simulink model "psk_demodulate_block1"  (R2020b)
settings: Solver=FixedStepDiscrete  StartTime=0.0  StopTime=10.0  RelTol=1e-3
settings Model: DataTypeOverride=Off  Creator=wardo  LastModifiedBy=wardo
settings DataIOCC: LimitDataPoints=on  SaveOutput=off  SaveTime=off
settings OptimizationCC: BlockReduction=off  ConditionallyExecuteInputs=off  DefaultParameterBehavior=Inlined  LifeSpan=inf
settings DebuggingCC: AlgebraicLoopMsg=error  SingleTaskRateTransMsg=error  AllowSymbolicDim=off  StrictBusMsg=ErrorOnBusTreatedAsVector  SFUnexpectedBacktrackingDiag=warning  SFNoUnconditionalDefaultTransitionDiag=warning  SFExecutionAtInitializationDiag=none  ArithmeticOperatorsInVariantConditions=warning
settings HardwareCC: ProdBitPerPointer=32  ProdBitPerSizeT=32  ProdBitPerPtrDiffT=32  ProdLargestAtomicFloat=None  ProdIntDivRoundTo=Undefined  ProdEndianess=Unspecified  ProdWordSize=32  ProdHWDeviceType=ASIC/FPGA->ASIC/FPGA  ProdEqTarget=off
settings SFSimCC: SimUseLocalCustomCode=off  CustomCodeUndefinedFunction=UseInterfaceOnly
settings RTWCC: RTWUseLocalCustomCode=off
settings CodeAppCC: StateflowObjectComments=on
settings GRTTargetCC: TargetLangStandard=C89/C90 (ANSI)
settings ConfigComp: CovScope=ReferencedModels  CovMetricSettings=dw  CovSaveCumulativeToWorkspaceVar=on  CovSaveSingleToWorkspaceVar=on  CovExternalEMLEnable=off  CovSFcnEnable=off

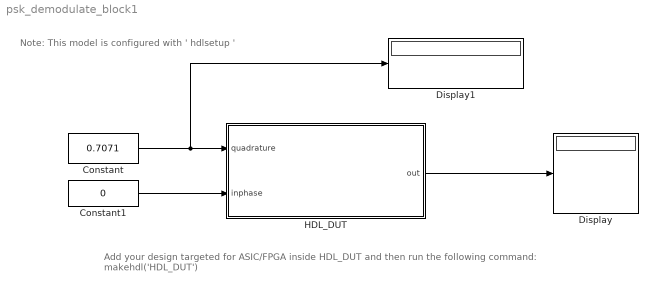
== system psk_demodulate_block1 ==
  note: Note: This model is configured with ' hdlsetup '
  note: Add your design targeted for ASIC/FPGA inside HDL_DUT and then run the following command:
      | makehdl('HDL_DUT')
  Constant : Constant  Value=0.7071  OutDataTypeStr=single  SampleTime=-1
  Constant1 : Constant  Value=0  OutDataTypeStr=single  SampleTime=-1
  Display : Display
  Display1 : Display
  HDL_DUT : Subsystem
  wires:
  Constant/1 -> Display1/1, HDL_DUT/1(quadrature)
  HDL_DUT/1(out) -> Display/1
  Constant1/1 -> HDL_DUT/2(inphase)

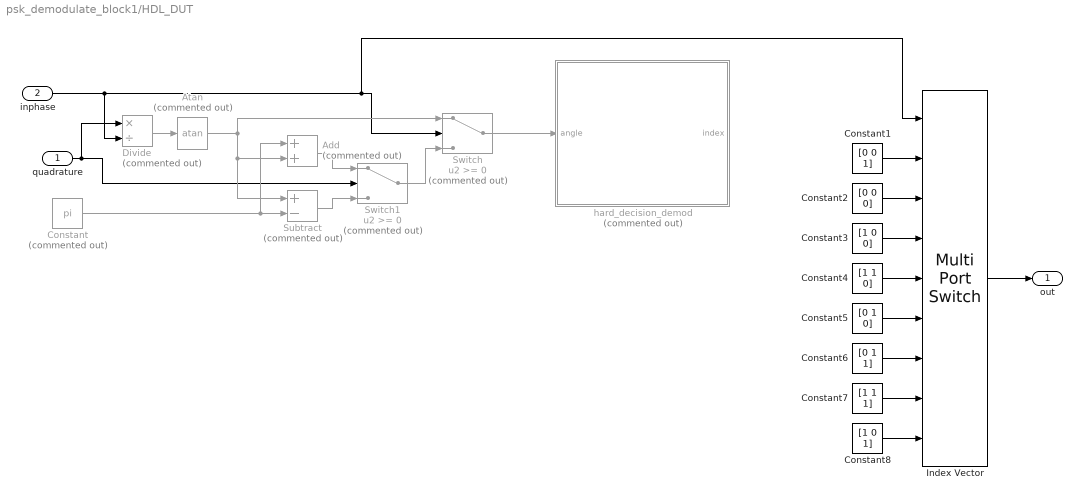
== system psk_demodulate_block1/HDL_DUT ==
  quadrature : Inport
  inphase : Inport  Port=2
  Add : Sum  Commented=on
  Atan : Trigonometry  Commented=on  Operator=atan  ApproximationMethod=CORDIC  OutputSignalType=real
  Constant : Constant  Commented=on  Value=pi  OutDataTypeStr=single  SampleTime=-1
  Constant1 : Constant  Value=[0 0 1]  OutDataTypeStr=single  SampleTime=-1
  Constant2 : Constant  Value=[0 0 0]  OutDataTypeStr=single  SampleTime=-1
  Constant3 : Constant  Value=[1 0 0]  OutDataTypeStr=single  SampleTime=-1
  Constant4 : Constant  Value=[1 1 0]  OutDataTypeStr=single  SampleTime=-1
  Constant5 : Constant  Value=[0 1 0]  OutDataTypeStr=single  SampleTime=-1
  Constant6 : Constant  Value=[0 1 1]  OutDataTypeStr=single  SampleTime=-1
  Constant7 : Constant  Value=[1 1 1]  OutDataTypeStr=single  SampleTime=-1
  Constant8 : Constant  Value=[1 0 1]  OutDataTypeStr=single  SampleTime=-1
  Divide : Product  Commented=on  Inputs=*/  SaturateOnIntegerOverflow=on
  Index Vector : MultiPortSwitch  Inputs=8  DataPortIndices={1,2,3,4,5,6,7,8}  DiagnosticForDefault=Warning  OutDataTypeStr=single
  Subtract : Sum  Commented=on  Inputs=+-
  Switch : Switch  Commented=on
  Switch1 : Switch  Commented=on
  hard_decision_demod : Subsystem  Commented=on
  out : Outport  VectorParamsAs1DForOutWhenUnconnected=off
  wires:
  Divide/1 -> Atan/1
  quadrature/1 -> Divide/1, Switch1/2
  inphase/1 -> Divide/2, Index Vector/1, Switch/2
  Atan/1 -> Add/2, Subtract/1, Switch/1
  Switch1/1 -> Switch/3
  Constant/1 -> Add/1, Subtract/2
  Add/1 -> Switch1/1
  Subtract/1 -> Switch1/3
  Index Vector/1 -> out/1
  Switch/1 -> hard_decision_demod/1(angle)
  Constant1/1 -> Index Vector/2
  Constant2/1 -> Index Vector/3
  Constant4/1 -> Index Vector/5
  Constant3/1 -> Index Vector/4
  Constant8/1 -> Index Vector/9
  Constant6/1 -> Index Vector/7
  Constant7/1 -> Index Vector/8
  Constant5/1 -> Index Vector/6

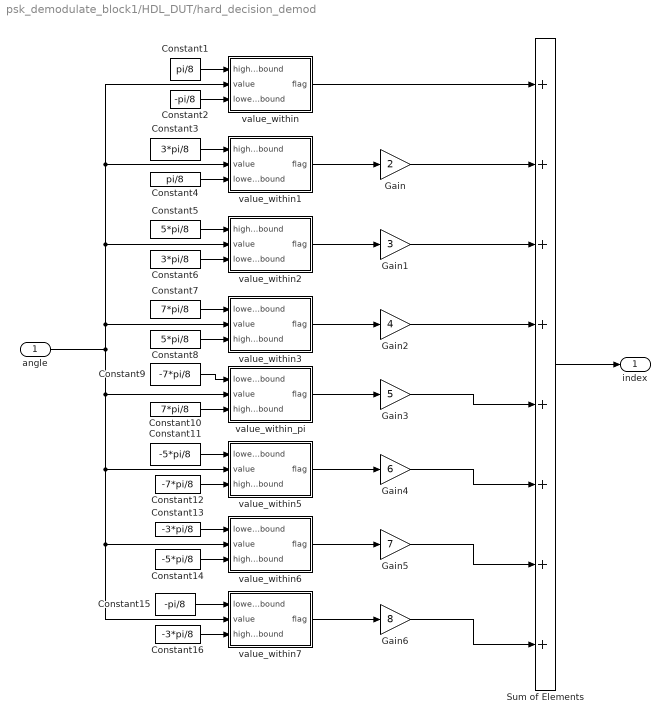
== system psk_demodulate_block1/HDL_DUT/hard_decision_demod ==
  angle : Inport
  Constant1 : Constant  Value=pi/8  OutDataTypeStr=single  SampleTime=-1
  Constant10 : Constant  Value=7*pi/8  OutDataTypeStr=single  SampleTime=-1
  Constant11 : Constant  Value=-5*pi/8  OutDataTypeStr=single  SampleTime=-1
  Constant12 : Constant  Value=-7*pi/8  OutDataTypeStr=single  SampleTime=-1
  Constant13 : Constant  Value=-3*pi/8  OutDataTypeStr=single  SampleTime=-1
  Constant14 : Constant  Value=-5*pi/8  OutDataTypeStr=single  SampleTime=-1
  Constant15 : Constant  Value=-pi/8  OutDataTypeStr=single  SampleTime=-1
  Constant16 : Constant  Value=-3*pi/8  OutDataTypeStr=single  SampleTime=-1
  Constant2 : Constant  Value=-pi/8  OutDataTypeStr=single  SampleTime=-1
  Constant3 : Constant  Value=3*pi/8  OutDataTypeStr=single  SampleTime=-1
  Constant4 : Constant  Value=pi/8  OutDataTypeStr=single  SampleTime=-1
  Constant5 : Constant  Value=5*pi/8  OutDataTypeStr=single  SampleTime=-1
  Constant6 : Constant  Value=3*pi/8  OutDataTypeStr=single  SampleTime=-1
  Constant7 : Constant  Value=7*pi/8  OutDataTypeStr=single  SampleTime=-1
  Constant8 : Constant  Value=5*pi/8  OutDataTypeStr=single  SampleTime=-1
  Constant9 : Constant  Value=-7*pi/8  OutDataTypeStr=single  SampleTime=-1
  Gain : Gain  Gain=2
  Gain1 : Gain  Gain=3
  Gain2 : Gain  Gain=4
  Gain3 : Gain  Gain=5
  Gain4 : Gain  Gain=6
  Gain5 : Gain  Gain=7
  Gain6 : Gain  Gain=8
  Sum of Elements : Sum  Inputs=++++++++
  value_within : Subsystem  TreatAsAtomicUnit=on
  value_within1 : Subsystem  TreatAsAtomicUnit=on
  value_within2 : Subsystem  TreatAsAtomicUnit=on
  value_within3 : Subsystem  TreatAsAtomicUnit=on
  value_within5 : Subsystem  TreatAsAtomicUnit=on
  value_within6 : Subsystem  TreatAsAtomicUnit=on
  value_within7 : Subsystem  TreatAsAtomicUnit=on
  value_within_pi : Subsystem  TreatAsAtomicUnit=on
  index : Outport
  wires:
  Constant2/1 -> value_within/3(lower_bound)
  Constant1/1 -> value_within/1(higher_bound)
  Sum of Elements/1 -> index/1
  Constant3/1 -> value_within1/1(higher_bound)
  Constant4/1 -> value_within1/3(lower_bound)
  Constant5/1 -> value_within2/1(higher_bound)
  Constant7/1 -> value_within3/1(lower_bound)
  Constant6/1 -> value_within2/3(lower_bound)
  Constant13/1 -> value_within6/1(lower_bound)
  Constant9/1 -> value_within_pi/1(lower_bound)
  Constant15/1 -> value_within7/1(lower_bound)
  Constant16/1 -> value_within7/3(higher_bound)
  Constant12/1 -> value_within5/3(higher_bound)
  Constant11/1 -> value_within5/1(lower_bound)
  Constant14/1 -> value_within6/3(higher_bound)
  Constant10/1 -> value_within_pi/3(higher_bound)
  angle/1 -> value_within1/2(value), value_within/2(value), value_within2/2(value), value_within3/2(value), value_within7/2(value), value_within6/2(value), value_within5/2(value), value_within_pi/2(value)
  value_within5/1(flag) -> Gain4/1
  value_within6/1(flag) -> Gain5/1
  value_within7/1(flag) -> Gain6/1
  value_within3/1(flag) -> Gain2/1
  value_within1/1(flag) -> Gain/1
  value_within/1(flag) -> Sum of Elements/1
  Gain/1 -> Sum of Elements/2
  value_within2/1(flag) -> Gain1/1
  Gain1/1 -> Sum of Elements/3
  Gain2/1 -> Sum of Elements/4
  value_within_pi/1(flag) -> Gain3/1
  Gain3/1 -> Sum of Elements/5
  Gain5/1 -> Sum of Elements/7
  Gain6/1 -> Sum of Elements/8
  Gain4/1 -> Sum of Elements/6
  Constant8/1 -> value_within3/3(higher_bound)

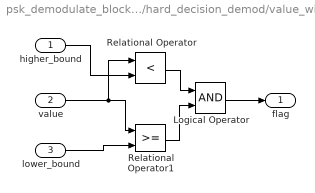
== system psk_demodulate_block1/HDL_DUT/hard_decision_demod/value_within ==
  higher_bound : Inport
  value : Inport  Port=2
  lower_bound : Inport  Port=3
  Logical Operator : Logic  AllPortsSameDT=off  OutDataTypeStr=boolean
  Relational Operator : RelationalOperator  Operator=<  OutDataTypeStr=boolean  RndMeth=Nearest
  Relational Operator1 : RelationalOperator  OutDataTypeStr=boolean  RndMeth=Nearest
  flag : Outport
  wires:
  value/1 -> Relational Operator/1, Relational Operator1/1
  Relational Operator/1 -> Logical Operator/1
  lower_bound/1 -> Relational Operator1/2
  Relational Operator1/1 -> Logical Operator/2
  Logical Operator/1 -> flag/1
  higher_bound/1 -> Relational Operator/2

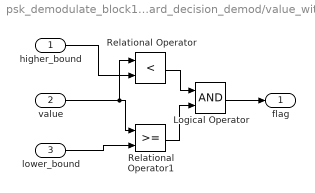
== system psk_demodulate_block1/HDL_DUT/hard_decision_demod/value_within1 ==
  higher_bound : Inport
  value : Inport  Port=2
  lower_bound : Inport  Port=3
  Logical Operator : Logic  AllPortsSameDT=off  OutDataTypeStr=boolean
  Relational Operator : RelationalOperator  Operator=<  OutDataTypeStr=boolean  RndMeth=Nearest
  Relational Operator1 : RelationalOperator  OutDataTypeStr=boolean  RndMeth=Nearest
  flag : Outport
  wires:
  value/1 -> Relational Operator/1, Relational Operator1/1
  Relational Operator/1 -> Logical Operator/1
  lower_bound/1 -> Relational Operator1/2
  Relational Operator1/1 -> Logical Operator/2
  Logical Operator/1 -> flag/1
  higher_bound/1 -> Relational Operator/2

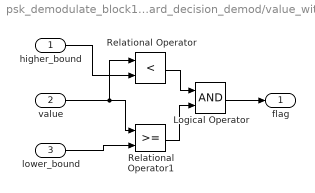
== system psk_demodulate_block1/HDL_DUT/hard_decision_demod/value_within2 ==
  higher_bound : Inport
  value : Inport  Port=2
  lower_bound : Inport  Port=3
  Logical Operator : Logic  AllPortsSameDT=off  OutDataTypeStr=boolean
  Relational Operator : RelationalOperator  Operator=<  OutDataTypeStr=boolean  RndMeth=Nearest
  Relational Operator1 : RelationalOperator  OutDataTypeStr=boolean  RndMeth=Nearest
  flag : Outport
  wires:
  value/1 -> Relational Operator/1, Relational Operator1/1
  Relational Operator/1 -> Logical Operator/1
  lower_bound/1 -> Relational Operator1/2
  Relational Operator1/1 -> Logical Operator/2
  Logical Operator/1 -> flag/1
  higher_bound/1 -> Relational Operator/2

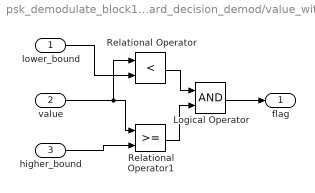
== system psk_demodulate_block1/HDL_DUT/hard_decision_demod/value_within3 ==
  lower_bound : Inport  OutDataTypeStr=single
  value : Inport  Port=2
  higher_bound : Inport  Port=3
  Logical Operator : Logic  AllPortsSameDT=off  OutDataTypeStr=boolean
  Relational Operator : RelationalOperator  Operator=<  OutDataTypeStr=boolean  RndMeth=Nearest
  Relational Operator1 : RelationalOperator  OutDataTypeStr=boolean  RndMeth=Nearest
  flag : Outport
  wires:
  value/1 -> Relational Operator/1, Relational Operator1/1
  Relational Operator/1 -> Logical Operator/1
  higher_bound/1 -> Relational Operator1/2
  Relational Operator1/1 -> Logical Operator/2
  Logical Operator/1 -> flag/1
  lower_bound/1 -> Relational Operator/2

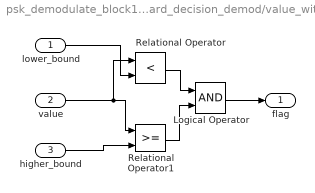
== system psk_demodulate_block1/HDL_DUT/hard_decision_demod/value_within5 ==
  lower_bound : Inport
  value : Inport  Port=2
  higher_bound : Inport  Port=3
  Logical Operator : Logic  AllPortsSameDT=off  OutDataTypeStr=boolean
  Relational Operator : RelationalOperator  Operator=<  OutDataTypeStr=boolean  RndMeth=Nearest
  Relational Operator1 : RelationalOperator  OutDataTypeStr=boolean  RndMeth=Nearest
  flag : Outport
  wires:
  lower_bound/1 -> Relational Operator/2
  value/1 -> Relational Operator1/1, Relational Operator/1
  Relational Operator/1 -> Logical Operator/1
  higher_bound/1 -> Relational Operator1/2
  Relational Operator1/1 -> Logical Operator/2
  Logical Operator/1 -> flag/1

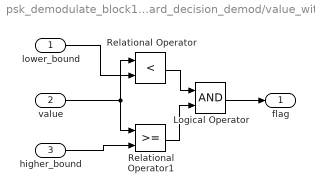
== system psk_demodulate_block1/HDL_DUT/hard_decision_demod/value_within6 ==
  lower_bound : Inport
  value : Inport  Port=2
  higher_bound : Inport  Port=3
  Logical Operator : Logic  AllPortsSameDT=off  OutDataTypeStr=boolean
  Relational Operator : RelationalOperator  Operator=<  OutDataTypeStr=boolean  RndMeth=Nearest
  Relational Operator1 : RelationalOperator  OutDataTypeStr=boolean  RndMeth=Nearest
  flag : Outport
  wires:
  value/1 -> Relational Operator1/1, Relational Operator/1
  Relational Operator/1 -> Logical Operator/1
  higher_bound/1 -> Relational Operator1/2
  Relational Operator1/1 -> Logical Operator/2
  Logical Operator/1 -> flag/1
  lower_bound/1 -> Relational Operator/2

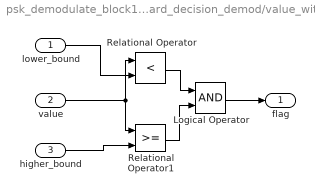
== system psk_demodulate_block1/HDL_DUT/hard_decision_demod/value_within7 ==
  lower_bound : Inport
  value : Inport  Port=2
  higher_bound : Inport  Port=3
  Logical Operator : Logic  AllPortsSameDT=off  OutDataTypeStr=boolean
  Relational Operator : RelationalOperator  Operator=<  OutDataTypeStr=boolean  RndMeth=Nearest
  Relational Operator1 : RelationalOperator  OutDataTypeStr=boolean  RndMeth=Nearest
  flag : Outport
  wires:
  value/1 -> Relational Operator/1, Relational Operator1/1
  Relational Operator/1 -> Logical Operator/1
  higher_bound/1 -> Relational Operator1/2
  Relational Operator1/1 -> Logical Operator/2
  Logical Operator/1 -> flag/1
  lower_bound/1 -> Relational Operator/2

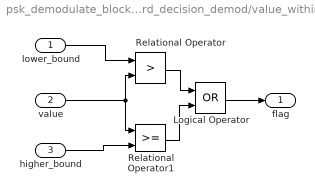
== system psk_demodulate_block1/HDL_DUT/hard_decision_demod/value_within_pi ==
  lower_bound : Inport
  value : Inport  Port=2
  higher_bound : Inport  Port=3
  Logical Operator : Logic  Operator=OR  AllPortsSameDT=off  OutDataTypeStr=boolean
  Relational Operator : RelationalOperator  Operator=>  OutDataTypeStr=boolean  RndMeth=Nearest
  Relational Operator1 : RelationalOperator  OutDataTypeStr=boolean  RndMeth=Nearest
  flag : Outport
  wires:
  lower_bound/1 -> Relational Operator/1
  value/1 -> Relational Operator1/1, Relational Operator/2
  Relational Operator/1 -> Logical Operator/1
  higher_bound/1 -> Relational Operator1/2
  Relational Operator1/1 -> Logical Operator/2
  Logical Operator/1 -> flag/1
